simulink model "Ejemplo_2"  (R2021b)
settings: Solver=VariableStepAuto  StartTime=0.0  StopTime=10.0  RelTol=1e-3
libraries: dspsrcs4 x6, commrandsrc3 x2, dsparch4 x2
settings Model: Creator=Hagui  LastModifiedBy=Hagui

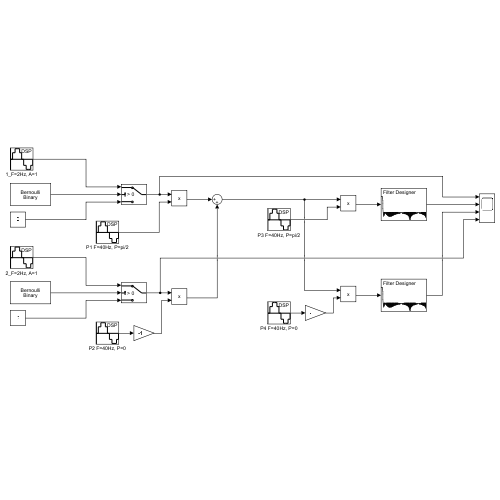
[thumbnail: Simulink's stored preview of the top-level diagram]
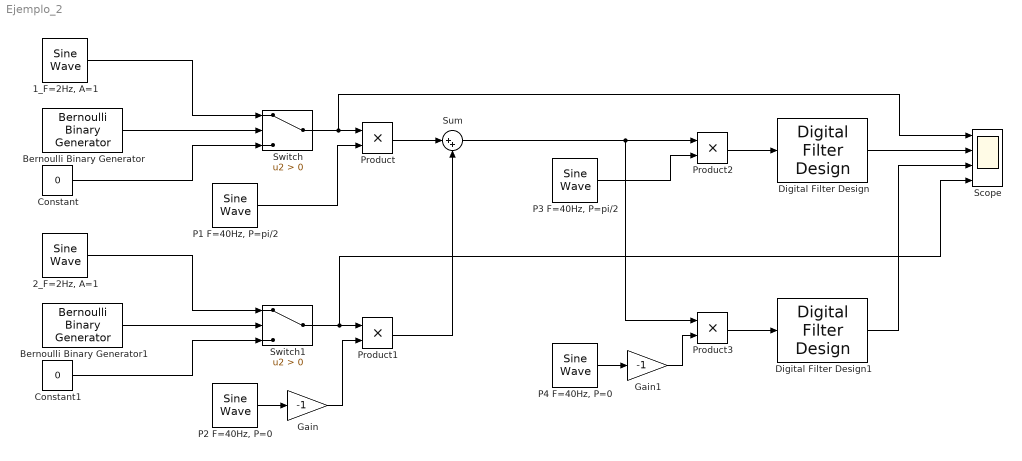
== system Ejemplo_2 ==
  "1_F=2Hz, A=1" : dspsrcs4/Sine Wave  Amplitude=1  Frequency=2  Phase=0  SampleMode=Discrete  OutComplex=Real  CompMethod=Trigonometric fcn  TableSize=Speed  SampleTime=1/1000  SamplesPerFrame=1  ResetState=Restart at time zero  OutputFrames=off  dataType=double  wordLen=16  udDataType=sfix(16)  fracBitsMode=Best precision  numFracBits=15  OutDataTypeStr=double  LastOutDataTypeStr=double
  "2_F=2Hz, A=1" : dspsrcs4/Sine Wave  Amplitude=1  Frequency=2  Phase=0  SampleMode=Discrete  OutComplex=Real  CompMethod=Trigonometric fcn  TableSize=Speed  SampleTime=1/1000  SamplesPerFrame=1  ResetState=Restart at time zero  OutputFrames=off  dataType=double  wordLen=16  udDataType=sfix(16)  fracBitsMode=Best precision  numFracBits=15  OutDataTypeStr=double  LastOutDataTypeStr=double
  Bernoulli Binary Generator : commrandsrc3/Bernoulli Binary Generator  ProbabilityOfZero=0.5  SeedSource=Auto  Seed=0  SampleTime=1  SamplesPerFrame=1  OutputDataType=double  SimulateUsing=Interpreted execution
  Bernoulli Binary Generator1 : commrandsrc3/Bernoulli Binary Generator  ProbabilityOfZero=0.5  SeedSource=Auto  Seed=0  SampleTime=1  SamplesPerFrame=1  OutputDataType=double  SimulateUsing=Interpreted execution
  Constant : Constant  Value=0
  Constant1 : Constant  Value=0
  Digital Filter Design : dsparch4/Digital Filter Design  mwdsp_browser_bugfix_var=off
  Digital Filter Design1 : dsparch4/Digital Filter Design  mwdsp_browser_bugfix_var=off
  Gain : Gain  Gain=-1
  Gain1 : Gain  Gain=-1
  "P1 F=40Hz, P=pi/2" : dspsrcs4/Sine Wave  Amplitude=1  Frequency=40  Phase=pi/2  SampleMode=Discrete  OutComplex=Real  CompMethod=Trigonometric fcn  TableSize=Speed  SampleTime=1/1000  SamplesPerFrame=1  ResetState=Restart at time zero  OutputFrames=off  dataType=double  wordLen=16  udDataType=sfix(16)  fracBitsMode=Best precision  numFracBits=15  OutDataTypeStr=double  LastOutDataTypeStr=double
  "P2 F=40Hz, P=0" : dspsrcs4/Sine Wave  Amplitude=1  Frequency=40  Phase=0  SampleMode=Discrete  OutComplex=Real  CompMethod=Trigonometric fcn  TableSize=Speed  SampleTime=1/1000  SamplesPerFrame=1  ResetState=Restart at time zero  OutputFrames=off  dataType=double  wordLen=16  udDataType=sfix(16)  fracBitsMode=Best precision  numFracBits=15  OutDataTypeStr=double  LastOutDataTypeStr=double
  "P3 F=40Hz, P=pi/2" : dspsrcs4/Sine Wave  Amplitude=1  Frequency=40  Phase=pi/2  SampleMode=Discrete  OutComplex=Real  CompMethod=Trigonometric fcn  TableSize=Speed  SampleTime=1/1000  SamplesPerFrame=1  ResetState=Restart at time zero  OutputFrames=off  dataType=double  wordLen=16  udDataType=sfix(16)  fracBitsMode=Best precision  numFracBits=15  OutDataTypeStr=double  LastOutDataTypeStr=double
  "P4 F=40Hz, P=0" : dspsrcs4/Sine Wave  Amplitude=1  Frequency=40  Phase=0  SampleMode=Discrete  OutComplex=Real  CompMethod=Trigonometric fcn  TableSize=Speed  SampleTime=1/1000  SamplesPerFrame=1  ResetState=Restart at time zero  OutputFrames=off  dataType=double  wordLen=16  udDataType=sfix(16)  fracBitsMode=Best precision  numFracBits=15  OutDataTypeStr=double  LastOutDataTypeStr=double
  Product{,1..3} (4 alike) : Product
  Scope : Scope  NumInputPorts=4
  Sum : Sum  Inputs=|++
  Switch : Switch  Criteria=u2 > Threshold
  Switch1 : Switch  Criteria=u2 > Threshold
  wires:
  Constant/1 -> Switch/3
  Bernoulli Binary Generator/1 -> Switch/2
  "1_F=2Hz, A=1"/1 -> Switch/1
  "2_F=2Hz, A=1"/1 -> Switch1/1
  Bernoulli Binary Generator1/1 -> Switch1/2
  Constant1/1 -> Switch1/3
  Switch/1 -> Scope/1, Product/1
  "P1 F=40Hz, P=pi/2"/1 -> Product/2
  Switch1/1 -> Scope/4, Product1/1
  "P2 F=40Hz, P=0"/1 -> Gain/1
  Gain/1 -> Product1/2
  Product/1 -> Sum/1
  Product1/1 -> Sum/2
  "P3 F=40Hz, P=pi/2"/1 -> Product2/2
  Sum/1 -> Product3/1, Product2/1
  "P4 F=40Hz, P=0"/1 -> Gain1/1
  Gain1/1 -> Product3/2
  Product3/1 -> Digital Filter Design1/1
  Product2/1 -> Digital Filter Design/1
  Digital Filter Design/1 -> Scope/2
  Digital Filter Design1/1 -> Scope/3
